simulink model "analiseLateroDirecional_NL"  (R2016a)
settings: Solver=ode4  StartTime=0.0  StopTime=300  FixedStep=0.01  RelTol=1e-3
undefined symbols (not defined in the file): Cphi, degtorad, Kp, Kphi, Kpsi, Kr, tau, Ue
libraries: simulink x2
settings Model: PauseTimes=20  Creator=Marcelo Henrique  LastModifiedBy=Marcelo
settings DataIOCC: LimitDataPoints=on  SaveFormat=Array
settings DebuggingCC: AlgebraicLoopMsg=none  UnderspecifiedInitializationDetection=Classic  MergeDetectMultiDrivingBlocksExec=none  StateNameClashWarn=warning
settings HardwareCC: ProdBitPerPointer=32  ProdLargestAtomicFloat=None  ProdIntDivRoundTo=Undefined  ProdEndianess=Unspecified  ProdWordSize=32  ProdHWDeviceType=32-bit Generic
settings ModelReferenceCC: PropagateSignalLabelsOutOfModel=off
settings ConfigComp: CovModelRefEnable=Off

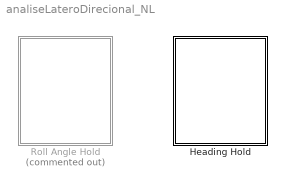
== system analiseLateroDirecional_NL ==
  Heading Hold : Subsystem
  Roll Angle Hold : Subsystem  Commented=on

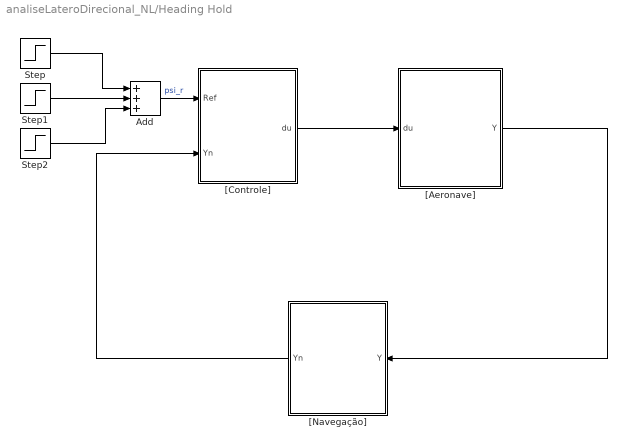
== system analiseLateroDirecional_NL/Heading Hold ==
  Add : Sum  Inputs=+++
  Step : Step  Time=50  After=degtorad(45)  SampleTime=0
  Step1 : Step  Time=150  After=degtorad(-90)  SampleTime=0
  Step2 : Step  Time=250  After=degtorad(45)  SampleTime=0
  "[Aeronave]" : Subsystem
  "[Controle]" : Subsystem
  "[Navegação]" : Subsystem
  wires:
  "[Aeronave]"/1(Y) -> "[Navegação]"/1(Y)
  "[Controle]"/1(du) -> "[Aeronave]"/1(du)
  "[Navegação]"/1(Yn) -> "[Controle]"/2(Yn)
  Step/1 -> Add/1
  Add/1 -> "[Controle]"/1(Ref)  "psi_r"
  Step1/1 -> Add/2
  Step2/1 -> Add/3

== system analiseLateroDirecional_NL/Roll Angle Hold ==
  Step : Step  Time=20  After=degtorad(20)  SampleTime=0
  "[Aeronave]" : Subsystem
  "[Controle]" : Subsystem
  "[Navegação]" : Subsystem
  wires:
  "[Aeronave]"/1(Y) -> "[Navegação]"/1(Y)
  "[Controle]"/1(du) -> "[Aeronave]"/1(du)
  "[Navegação]"/1(Yn) -> "[Controle]"/2(Yn)
  Step/1 -> "[Controle]"/1(Ref)  "phi_r"

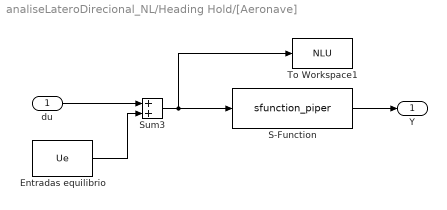
== system analiseLateroDirecional_NL/Heading Hold/[Aeronave] ==
  du : Inport
  Entradas equilibrio : Constant  Value=Ue
  S-Function : S-Function  FunctionName=sfunction_piper  Parameters=par_gen,par_aero,par_prop, Xe  SFunctionDeploymentMode=off  EnableBusSupport=off
  Sum3 : Sum
  To Workspace1 : ToWorkspace  VariableName=NLU  SaveFormat=Timeseries  SampleTime=-1
  Y : Outport
  wires:
  du/1 -> Sum3/1
  Sum3/1 -> S-Function/1, To Workspace1/1
  S-Function/1 -> Y/1
  Entradas equilibrio/1 -> Sum3/2

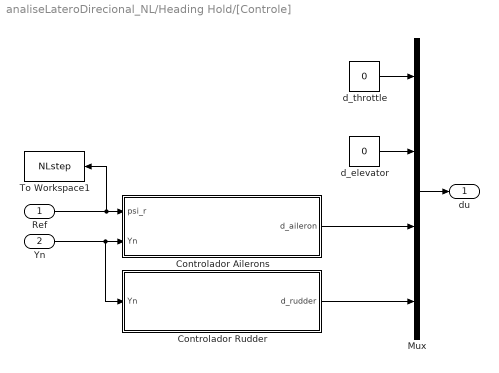
== system analiseLateroDirecional_NL/Heading Hold/[Controle] ==
  Ref : Inport
  Yn : Inport  Port=2
  Controlador Ailerons : Subsystem
  Controlador Rudder : Subsystem
  Mux : Mux
  To Workspace1 : ToWorkspace  VariableName=NLstep  SaveFormat=Timeseries  SampleTime=-1
  d_elevator : Constant  Value=0
  d_throttle : Constant  Value=0
  du : Outport
  wires:
  Yn/1 -> Controlador Rudder/1(Yn), Controlador Ailerons/2(Yn)
  Mux/1 -> du/1
  Ref/1 -> To Workspace1/1, Controlador Ailerons/1(psi_r)
  Controlador Ailerons/1(d_aileron) -> Mux/3
  d_throttle/1 -> Mux/1
  d_elevator/1 -> Mux/2
  Controlador Rudder/1(d_rudder) -> Mux/4

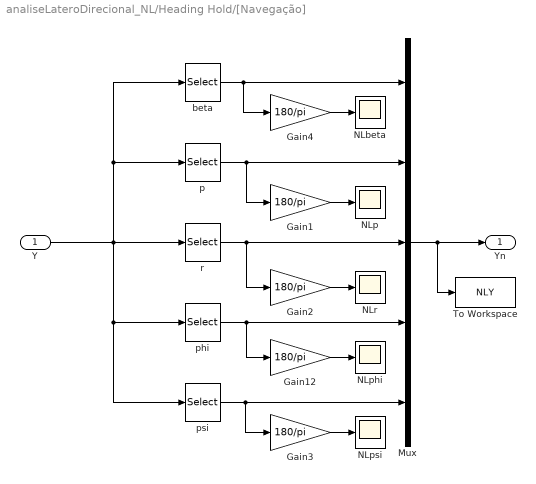
== system analiseLateroDirecional_NL/Heading Hold/[Navegação] ==
  Y : Inport
  Gain{1..4,12} (5 alike) : Gain  Gain=180/pi
  Mux : Mux  Inputs=5
  NLbeta : Scope
  NLp : Scope
  NLphi : Scope
  NLpsi : Scope
  NLr : Scope
  To Workspace : ToWorkspace  VariableName=NLY  SaveFormat=Timeseries  SampleTime=-1
  beta : Selector  InputPortWidth=12  IndexOptions=Index vector (dialog)  Indices=[3]  OutputSizes=1
  p : Selector  InputPortWidth=12  IndexOptions=Index vector (dialog)  Indices=[4]  OutputSizes=1
  phi : Selector  InputPortWidth=12  IndexOptions=Index vector (dialog)  Indices=[7]  OutputSizes=1
  psi : Selector  InputPortWidth=12  IndexOptions=Index vector (dialog)  Indices=[9]  OutputSizes=1
  r : Selector  InputPortWidth=12  IndexOptions=Index vector (dialog)  Indices=[6]  OutputSizes=1
  Yn : Outport
  wires:
  Y/1 -> psi/1, phi/1, beta/1, p/1, r/1
  Gain12/1 -> NLphi/1
  beta/1 -> Gain4/1, Mux/1
  phi/1 -> Gain12/1, Mux/4
  psi/1 -> Gain3/1, Mux/5
  Gain1/1 -> NLp/1
  p/1 -> Gain1/1, Mux/2
  Gain2/1 -> NLr/1
  r/1 -> Gain2/1, Mux/3
  Mux/1 -> To Workspace/1, Yn/1
  Gain3/1 -> NLpsi/1
  Gain4/1 -> NLbeta/1

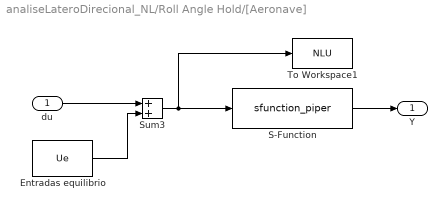
== system analiseLateroDirecional_NL/Roll Angle Hold/[Aeronave] ==
  du : Inport
  Entradas equilibrio : Constant  Value=Ue
  S-Function : S-Function  FunctionName=sfunction_piper  Parameters=par_gen,par_aero,par_prop, Xe  SFunctionDeploymentMode=off  EnableBusSupport=off
  Sum3 : Sum
  To Workspace1 : ToWorkspace  VariableName=NLU  SaveFormat=Timeseries  SampleTime=-1
  Y : Outport
  wires:
  du/1 -> Sum3/1
  Sum3/1 -> S-Function/1, To Workspace1/1
  S-Function/1 -> Y/1
  Entradas equilibrio/1 -> Sum3/2

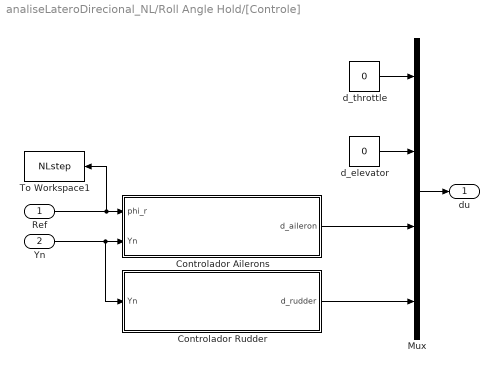
== system analiseLateroDirecional_NL/Roll Angle Hold/[Controle] ==
  Ref : Inport
  Yn : Inport  Port=2
  Controlador Ailerons : Subsystem
  Controlador Rudder : Subsystem
  Mux : Mux
  To Workspace1 : ToWorkspace  VariableName=NLstep  SaveFormat=Timeseries  SampleTime=-1
  d_elevator : Constant  Value=0
  d_throttle : Constant  Value=0
  du : Outport
  wires:
  Yn/1 -> Controlador Rudder/1(Yn), Controlador Ailerons/2(Yn)
  Mux/1 -> du/1
  Ref/1 -> To Workspace1/1, Controlador Ailerons/1(phi_r)
  Controlador Ailerons/1(d_aileron) -> Mux/3
  d_throttle/1 -> Mux/1
  d_elevator/1 -> Mux/2
  Controlador Rudder/1(d_rudder) -> Mux/4

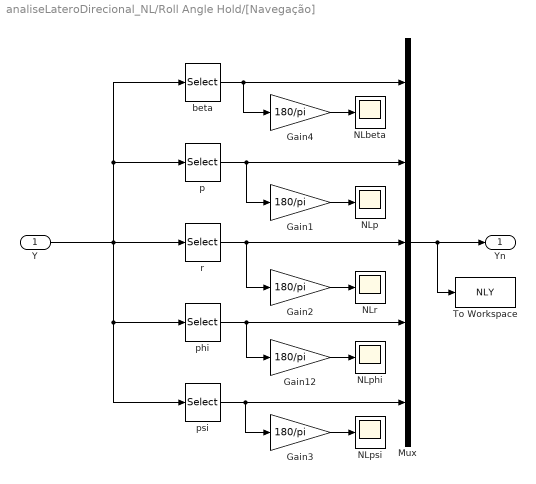
== system analiseLateroDirecional_NL/Roll Angle Hold/[Navegação] ==
  Y : Inport
  Gain{1..4,12} (5 alike) : Gain  Gain=180/pi
  Mux : Mux  Inputs=5
  NLbeta : Scope
  NLp : Scope
  NLphi : Scope
  NLpsi : Scope
  NLr : Scope
  To Workspace : ToWorkspace  VariableName=NLY  SaveFormat=Timeseries  SampleTime=-1
  beta : Selector  InputPortWidth=12  IndexOptions=Index vector (dialog)  Indices=[3]  OutputSizes=1
  p : Selector  InputPortWidth=12  IndexOptions=Index vector (dialog)  Indices=[4]  OutputSizes=1
  phi : Selector  InputPortWidth=12  IndexOptions=Index vector (dialog)  Indices=[7]  OutputSizes=1
  psi : Selector  InputPortWidth=12  IndexOptions=Index vector (dialog)  Indices=[9]  OutputSizes=1
  r : Selector  InputPortWidth=12  IndexOptions=Index vector (dialog)  Indices=[6]  OutputSizes=1
  Yn : Outport
  wires:
  Y/1 -> psi/1, phi/1, beta/1, p/1, r/1
  Gain12/1 -> NLphi/1
  beta/1 -> Gain4/1, Mux/1
  phi/1 -> Gain12/1, Mux/4
  psi/1 -> Gain3/1, Mux/5
  Gain1/1 -> NLp/1
  p/1 -> Gain1/1, Mux/2
  Gain2/1 -> NLr/1
  r/1 -> Gain2/1, Mux/3
  Mux/1 -> To Workspace/1, Yn/1
  Gain3/1 -> NLpsi/1
  Gain4/1 -> NLbeta/1

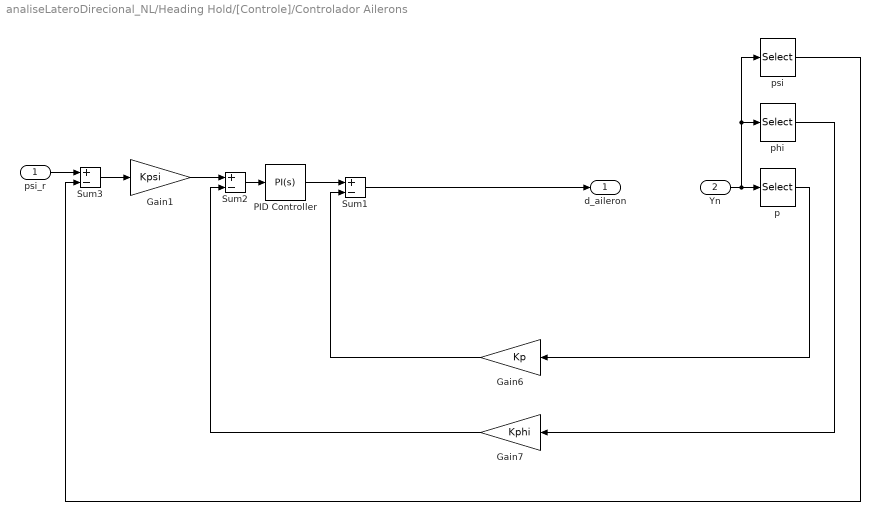
== system analiseLateroDirecional_NL/Heading Hold/[Controle]/Controlador Ailerons ==
  psi_r : Inport
  Yn : Inport  Port=2
  Gain1 : Gain  Gain=Kpsi
  Gain6 : Gain  Gain=Kp
  Gain7 : Gain  Gain=Kphi
  PID Controller : simulink/Continuous/PID Controller  Controller=PI  TimeDomain=Continuous-time  SampleTime=-1  IntegratorMethod=Forward Euler  FilterMethod=Forward Euler  Form=Parallel  UseFilter=on  ControllerParametersSource=internal  P=Cphi.Kp  I=Cphi.Ki  D=0  N=100  InitialConditionSource=internal  InitialConditionForIntegrator=0  InitialConditionForFilter=0  ExternalReset=none  LimitOutput=off  UpperSaturationLimit=inf  LowerSaturationLimit=-inf  LinearizeAsGain=on  AntiWindupMode=none  Kb=1  TrackingMode=off  Kt=1  PParamMin=[]  PParamMax=[]  IParamMin=[]  IParamMax=[]  DParamMin=[]  DParamMax=[]  NParamMin=[]  NParamMax=[]  KbParamMin=[]  KbParamMax=[]  KtParamMin=[]  KtParamMax=[]  POutMin=[]  POutMax=[]  IOutMin=[]  IOutMax=[]  DOutMin=[]  DOutMax=[]  NOutMin=[]  NOutMax=[]  KbOutMin=[]  KbOutMax=[]  KtOutMin=[]  KtOutMax=[]  IntegratorOutMin=[]  IntegratorOutMax=[]  FilterOutMin=[]  FilterOutMax=[]  SumOutMin=[]  SumOutMax=[]  SumI1OutMin=[]  SumI1OutMax=[]  SumI2OutMin=[]  SumI2OutMax=[]  SumI3OutMin=[]  SumI3OutMax=[]  SumDOutMin=[]  SumDOutMax=[]  SaturationOutMin=[]  SaturationOutMax=[]  IntegratorContinuousStateAttributes=''  IntegratorStateMustResolveToSignalObject=off  IntegratorRTWStateStorageClass=Auto  FilterContinuousStateAttributes=''  FilterStateMustResolveToSignalObject=off  FilterRTWStateStorageClass=Auto  DifferentiatorICPrevScaledInput=0  DifferentiatorOutMin=[]  DifferentiatorOutMax=[]
  Sum1 : Sum  Inputs=+-
  Sum2 : Sum  Inputs=+-
  Sum3 : Sum  Inputs=+-
  p : Selector  InputPortWidth=5  IndexOptions=Index vector (dialog)  Indices=[2]  OutputSizes=1
  phi : Selector  InputPortWidth=5  IndexOptions=Index vector (dialog)  Indices=[4]  OutputSizes=1
  psi : Selector  InputPortWidth=5  IndexOptions=Index vector (dialog)  Indices=[5]  OutputSizes=1
  d_aileron : Outport
  wires:
  phi/1 -> Gain7/1
  p/1 -> Gain6/1
  Gain6/1 -> Sum1/2
  Gain7/1 -> Sum2/2
  PID Controller/1 -> Sum1/1
  Sum2/1 -> PID Controller/1
  Yn/1 -> psi/1, phi/1, p/1
  Sum1/1 -> d_aileron/1
  psi_r/1 -> Sum3/1
  Gain1/1 -> Sum2/1
  Sum3/1 -> Gain1/1
  psi/1 -> Sum3/2

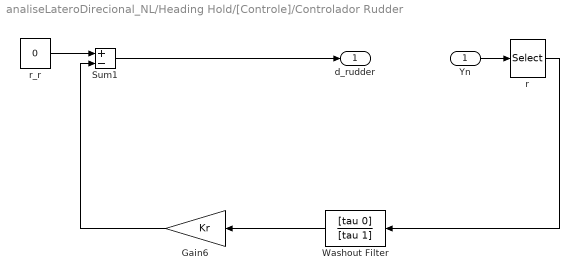
== system analiseLateroDirecional_NL/Heading Hold/[Controle]/Controlador Rudder ==
  Yn : Inport
  Gain6 : Gain  Gain=Kr
  Sum1 : Sum  Inputs=+-
  Washout Filter : TransferFcn  Numerator=[tau 0]  Denominator=[tau 1]
  r : Selector  InputPortWidth=5  IndexOptions=Index vector (dialog)  Indices=[3]  OutputSizes=1
  r_r : Constant  Value=0
  d_rudder : Outport
  wires:
  r/1 -> Washout Filter/1
  Gain6/1 -> Sum1/2
  r_r/1 -> Sum1/1
  Yn/1 -> r/1
  Sum1/1 -> d_rudder/1
  Washout Filter/1 -> Gain6/1

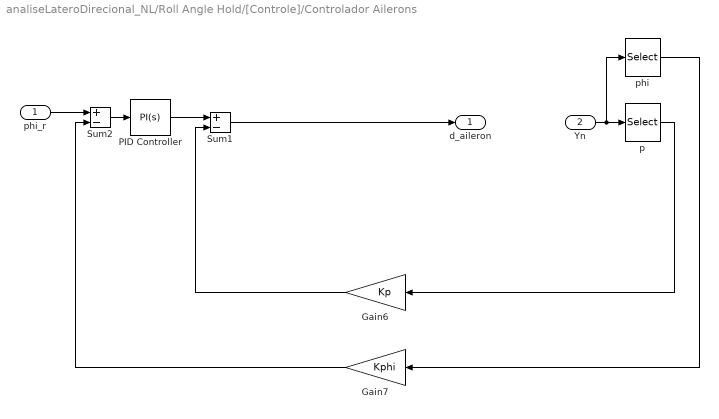
== system analiseLateroDirecional_NL/Roll Angle Hold/[Controle]/Controlador Ailerons ==
  phi_r : Inport
  Yn : Inport  Port=2
  Gain6 : Gain  Gain=Kp
  Gain7 : Gain  Gain=Kphi
  PID Controller : simulink/Continuous/PID Controller  Controller=PI  TimeDomain=Continuous-time  SampleTime=-1  IntegratorMethod=Forward Euler  FilterMethod=Forward Euler  Form=Parallel  UseFilter=on  ControllerParametersSource=internal  P=Cphi.Kp  I=Cphi.Ki  D=0  N=100  InitialConditionSource=internal  InitialConditionForIntegrator=0  InitialConditionForFilter=0  ExternalReset=none  ZeroCross=off  LimitOutput=off  UpperSaturationLimit=inf  LowerSaturationLimit=-inf  LinearizeAsGain=on  AntiWindupMode=none  Kb=1  TrackingMode=off  Kt=1  PParamMin=[]  PParamMax=[]  IParamMin=[]  IParamMax=[]  DParamMin=[]  DParamMax=[]  NParamMin=[]  NParamMax=[]  KbParamMin=[]  KbParamMax=[]  KtParamMin=[]  KtParamMax=[]  POutMin=[]  POutMax=[]  IOutMin=[]  IOutMax=[]  DOutMin=[]  DOutMax=[]  NOutMin=[]  NOutMax=[]  KbOutMin=[]  KbOutMax=[]  KtOutMin=[]  KtOutMax=[]  IntegratorOutMin=[]  IntegratorOutMax=[]  FilterOutMin=[]  FilterOutMax=[]  SumOutMin=[]  SumOutMax=[]  SumI1OutMin=[]  SumI1OutMax=[]  SumI2OutMin=[]  SumI2OutMax=[]  SumI3OutMin=[]  SumI3OutMax=[]  SumDOutMin=[]  SumDOutMax=[]  SaturationOutMin=[]  SaturationOutMax=[]  IntegratorContinuousStateAttributes=''  IntegratorStateMustResolveToSignalObject=off  IntegratorRTWStateStorageClass=Auto  FilterContinuousStateAttributes=''  FilterStateMustResolveToSignalObject=off  FilterRTWStateStorageClass=Auto  DifferentiatorICPrevScaledInput=0  DifferentiatorOutMin=[]  DifferentiatorOutMax=[]
  Sum1 : Sum  Inputs=+-
  Sum2 : Sum  Inputs=+-
  p : Selector  InputPortWidth=5  IndexOptions=Index vector (dialog)  Indices=[2]  OutputSizes=1
  phi : Selector  InputPortWidth=5  IndexOptions=Index vector (dialog)  Indices=[4]  OutputSizes=1
  d_aileron : Outport
  wires:
  phi/1 -> Gain7/1
  p/1 -> Gain6/1
  Gain6/1 -> Sum1/2
  Gain7/1 -> Sum2/2
  PID Controller/1 -> Sum1/1
  Sum2/1 -> PID Controller/1
  Yn/1 -> phi/1, p/1
  Sum1/1 -> d_aileron/1
  phi_r/1 -> Sum2/1

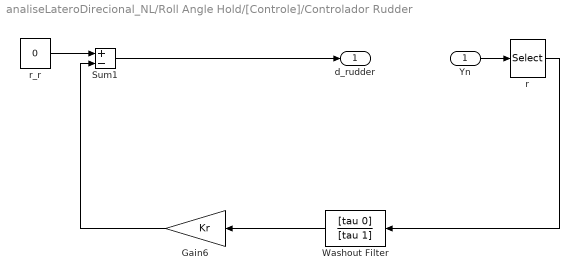
== system analiseLateroDirecional_NL/Roll Angle Hold/[Controle]/Controlador Rudder ==
  Yn : Inport
  Gain6 : Gain  Gain=Kr
  Sum1 : Sum  Inputs=+-
  Washout Filter : TransferFcn  Numerator=[tau 0]  Denominator=[tau 1]
  r : Selector  InputPortWidth=5  IndexOptions=Index vector (dialog)  Indices=[3]  OutputSizes=1
  r_r : Constant  Value=0
  d_rudder : Outport
  wires:
  r/1 -> Washout Filter/1
  Gain6/1 -> Sum1/2
  r_r/1 -> Sum1/1
  Yn/1 -> r/1
  Sum1/1 -> d_rudder/1
  Washout Filter/1 -> Gain6/1
